simulink model "mba_model"  (R2016a)
settings: Solver=VariableStepAuto  StartTime=0.0  StopTime=1  RelTol=1e-5
settings Model: Creator=manuel  LastModifiedBy=manuel

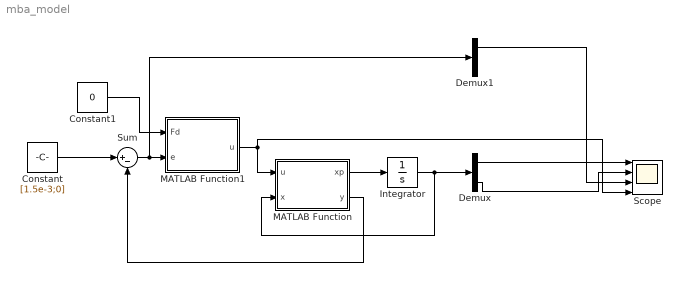
== system mba_model ==
  Constant : Constant  Value=[1.5e-3;0]
  Constant1 : Constant  Value=0
  Demux : Demux  Outputs=3
  Demux1 : Demux  Outputs=2
  Integrator : Integrator  InitialCondition=[1.8e-3;0;.25]  LimitOutput=on  UpperSaturationLimit=[3e-3;inf;5]  LowerSaturationLimit=[.8e-3;-inf;-0.5]
  MATLAB Function : MATLAB Function  TreatAsAtomicUnit=on
  MATLAB Function1 : MATLAB Function  TreatAsAtomicUnit=on
  Scope : Scope  NumInputPorts=4
  Sum : Sum  Inputs=|+-
  wires:
  MATLAB Function/1(xp) -> Integrator/1
  Constant/1 -> Sum/1
  MATLAB Function/2(y) -> Sum/2
  Sum/1 -> Demux1/1, MATLAB Function1/2(e)
  MATLAB Function1/1(u) -> MATLAB Function/1(u), Scope/4
  Constant1/1 -> MATLAB Function1/1(Fd)
  Integrator/1 -> Demux/1, MATLAB Function/2(x)
  Demux/1 -> Scope/1
  Demux/3 -> Scope/2
  Demux1/1 -> Scope/3

== matlab function mba_model/MATLAB Function1 ==
  data: Fd input; e input; u output
function u = controller(Fd,e)
%#codegen

k = [-10000,-1000];
v = k*e;
if(v < -24)
   v = -24;
elseif(v > 24)
   v = 24;
end
u = [Fd;v];

== matlab function mba_model/MATLAB Function ==
  data: u input; x input; xp output; y output
function [xp,y] = mba_ss(u,x)
%#codegen
m = .1;
[F,Vfem,R,L] = get_electromagnet_parameters(x(1),x(2),x(3));

xp = [  x(2);
        (u(1)+F+(9.8*m))/m;
        ((u(2)-Vfem-(x(3)*R))/L)];

y = [x(1);x(2)];
